simulink model "Hornsea_anant_with_STATCOM (1)"  (R2023b)
settings: Solver=ode1  StartTime=0.0  StopTime=sim_config.Tsim  RelTol=1e-3
undefined symbols (not defined in the file): sim_config
libraries: myLibrary x43, spsThreePhaseVIMeasurementLib x22, spsPower3phInstantaneousLib x11, spspowerguiLib x1
settings Model: Creator=Josep  LastModifiedBy=Josep

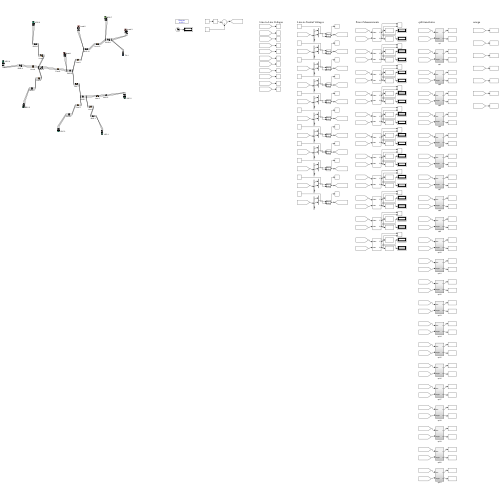
[thumbnail: Simulink's stored preview of the top-level diagram]
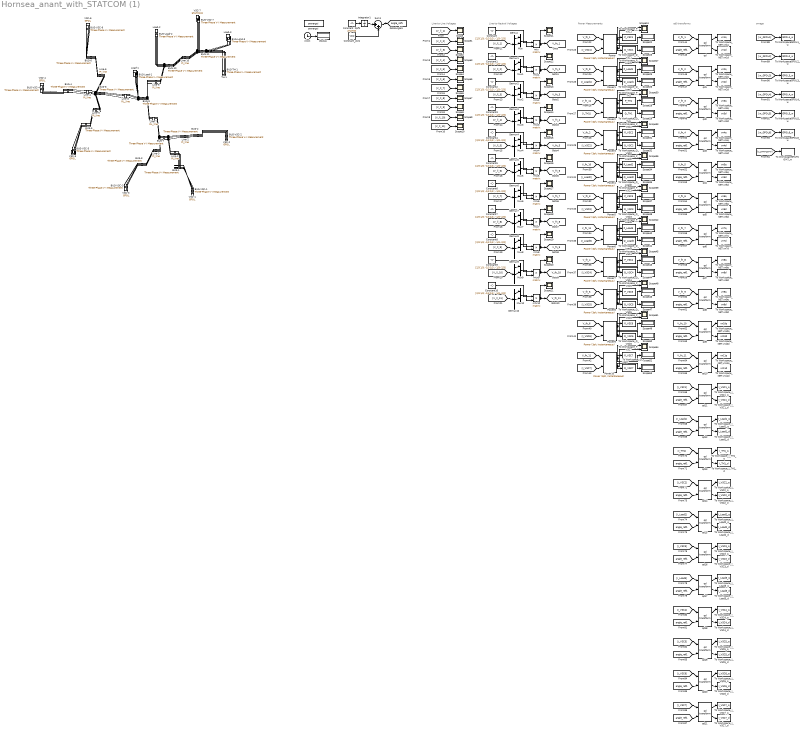
== system Hornsea_anant_with_STATCOM (1) ==
  note: Line-to-Line Voltages
  note: Line-to-Neutral Voltages
  note: Power Measurements
  note: qd0 transforms
  note: omega
  BUS-1 : spsThreePhaseVIMeasurementLib/Three-Phase V-I Measurement  VoltageMeasurement=phase-to-phase  SetLabelV=on  LabelV=V_ll_1  Vpu=off  VpuLL=off  CurrentMeasurement=yes  SetLabelI=on  LabelI=I_1  Ipu=off  Pbase=100e6  Vbase=500e3  OutputType=Complex  PhasorSimulation=off  PSBequivalent=0
  BUS-10 : spsThreePhaseVIMeasurementLib/Three-Phase V-I Measurement  VoltageMeasurement=phase-to-phase  SetLabelV=on  LabelV=V_ll_10  Vpu=off  VpuLL=off  CurrentMeasurement=yes  SetLabelI=on  LabelI=I_10  Ipu=off  Pbase=100e6  Vbase=500e3  OutputType=Complex  PhasorSimulation=off  PSBequivalent=0
  BUS-11 : spsThreePhaseVIMeasurementLib/Three-Phase V-I Measurement  VoltageMeasurement=phase-to-phase  SetLabelV=on  LabelV=V_ll_11  Vpu=off  VpuLL=off  CurrentMeasurement=yes  SetLabelI=on  LabelI=I_11  Ipu=off  Pbase=100e6  Vbase=500e3  OutputType=Complex  PhasorSimulation=off  PSBequivalent=0
  BUS-2 : spsThreePhaseVIMeasurementLib/Three-Phase V-I Measurement  VoltageMeasurement=phase-to-phase  SetLabelV=on  LabelV=V_ll_2  Vpu=off  VpuLL=off  CurrentMeasurement=yes  SetLabelI=on  LabelI=I_2  Ipu=off  Pbase=100e6  Vbase=500e3  OutputType=Complex  PhasorSimulation=off  PSBequivalent=0
  BUS-3 : spsThreePhaseVIMeasurementLib/Three-Phase V-I Measurement  VoltageMeasurement=phase-to-phase  SetLabelV=on  LabelV=V_ll_3  Vpu=off  VpuLL=off  CurrentMeasurement=yes  SetLabelI=on  LabelI=I_3  Ipu=off  Pbase=100e6  Vbase=500e3  OutputType=Complex  PhasorSimulation=off  PSBequivalent=0
  BUS-4 : spsThreePhaseVIMeasurementLib/Three-Phase V-I Measurement  VoltageMeasurement=phase-to-phase  SetLabelV=on  LabelV=V_ll_4  Vpu=off  VpuLL=off  CurrentMeasurement=yes  SetLabelI=on  LabelI=I_4  Ipu=off  Pbase=100e6  Vbase=500e3  OutputType=Complex  PhasorSimulation=off  PSBequivalent=0
  BUS-5 : spsThreePhaseVIMeasurementLib/Three-Phase V-I Measurement  VoltageMeasurement=phase-to-phase  SetLabelV=on  LabelV=V_ll_5  Vpu=off  VpuLL=off  CurrentMeasurement=yes  SetLabelI=on  LabelI=I_5  Ipu=off  Pbase=100e6  Vbase=500e3  OutputType=Complex  PhasorSimulation=off  PSBequivalent=0
  BUS-6 : spsThreePhaseVIMeasurementLib/Three-Phase V-I Measurement  VoltageMeasurement=phase-to-phase  SetLabelV=on  LabelV=V_ll_6  Vpu=off  VpuLL=off  CurrentMeasurement=yes  SetLabelI=on  LabelI=I_6  Ipu=off  Pbase=100e6  Vbase=500e3  OutputType=Complex  PhasorSimulation=off  PSBequivalent=0
  BUS-7 : spsThreePhaseVIMeasurementLib/Three-Phase V-I Measurement  VoltageMeasurement=phase-to-phase  SetLabelV=on  LabelV=V_ll_7  Vpu=off  VpuLL=off  CurrentMeasurement=yes  SetLabelI=on  LabelI=I_7  Ipu=off  Pbase=100e6  Vbase=500e3  OutputType=Complex  PhasorSimulation=off  PSBequivalent=0
  BUS-8 : spsThreePhaseVIMeasurementLib/Three-Phase V-I Measurement  VoltageMeasurement=phase-to-phase  SetLabelV=on  LabelV=V_ll_8  Vpu=off  VpuLL=off  CurrentMeasurement=yes  SetLabelI=on  LabelI=I_8  Ipu=off  Pbase=100e6  Vbase=500e3  OutputType=Complex  PhasorSimulation=off  PSBequivalent=0
  BUS-9 : spsThreePhaseVIMeasurementLib/Three-Phase V-I Measurement  VoltageMeasurement=phase-to-phase  SetLabelV=on  LabelV=V_ll_9  Vpu=off  VpuLL=off  CurrentMeasurement=yes  SetLabelI=on  LabelI=I_9  Ipu=off  Pbase=100e6  Vbase=500e3  OutputType=Complex  PhasorSimulation=off  PSBequivalent=0
  BUS-Load-1 : spsThreePhaseVIMeasurementLib/Three-Phase V-I Measurement  VoltageMeasurement=phase-to-phase  SetLabelV=on  LabelV=V_Load_1  Vpu=off  VpuLL=off  CurrentMeasurement=yes  SetLabelI=on  LabelI=I_Load1  Ipu=off  Pbase=100e6  Vbase=500e3  OutputType=Complex  PhasorSimulation=off  PSBequivalent=0
  BUS-Load-2 : spsThreePhaseVIMeasurementLib/Three-Phase V-I Measurement  VoltageMeasurement=phase-to-phase  SetLabelV=on  LabelV=V_Load_2  Vpu=off  VpuLL=off  CurrentMeasurement=yes  SetLabelI=on  LabelI=I_Load2  Ipu=off  Pbase=100e6  Vbase=500e3  OutputType=Complex  PhasorSimulation=off  PSBequivalent=0
  BUS-Load-3 : spsThreePhaseVIMeasurementLib/Three-Phase V-I Measurement  VoltageMeasurement=phase-to-phase  SetLabelV=on  LabelV=V_Load_3  Vpu=off  VpuLL=off  CurrentMeasurement=yes  SetLabelI=on  LabelI=I_Load3  Ipu=off  Pbase=100e6  Vbase=500e3  OutputType=Complex  PhasorSimulation=off  PSBequivalent=0
  BUS-TH-1 : spsThreePhaseVIMeasurementLib/Three-Phase V-I Measurement  VoltageMeasurement=phase-to-phase  SetLabelV=on  LabelV=V_TH_1  Vpu=off  VpuLL=off  CurrentMeasurement=yes  SetLabelI=on  LabelI=I_TH1  Ipu=off  Pbase=100e6  Vbase=500e3  OutputType=Complex  PhasorSimulation=off  PSBequivalent=0
  BUS-VSC-1 : spsThreePhaseVIMeasurementLib/Three-Phase V-I Measurement  VoltageMeasurement=phase-to-phase  SetLabelV=on  LabelV=V_VSC_1  Vpu=off  VpuLL=off  CurrentMeasurement=yes  SetLabelI=on  LabelI=I_VSC1  Ipu=off  Pbase=100e6  Vbase=500e3  OutputType=Complex  PhasorSimulation=off  PSBequivalent=0
  BUS-VSC-2 : spsThreePhaseVIMeasurementLib/Three-Phase V-I Measurement  VoltageMeasurement=phase-to-phase  SetLabelV=on  LabelV=V_VSC_2  Vpu=off  VpuLL=off  CurrentMeasurement=yes  SetLabelI=on  LabelI=I_VSC2  Ipu=off  Pbase=100e6  Vbase=500e3  OutputType=Complex  PhasorSimulation=off  PSBequivalent=0
  BUS-VSC-3 : spsThreePhaseVIMeasurementLib/Three-Phase V-I Measurement  VoltageMeasurement=phase-to-phase  SetLabelV=on  LabelV=V_VSC_3  Vpu=off  VpuLL=off  CurrentMeasurement=yes  SetLabelI=on  LabelI=I_VSC3  Ipu=off  Pbase=100e6  Vbase=500e3  OutputType=Complex  PhasorSimulation=off  PSBequivalent=0
  BUS-VSC-4 : spsThreePhaseVIMeasurementLib/Three-Phase V-I Measurement  VoltageMeasurement=phase-to-phase  SetLabelV=on  LabelV=V_VSC_4  Vpu=off  VpuLL=off  CurrentMeasurement=yes  SetLabelI=on  LabelI=I_VSC4  Ipu=off  Pbase=100e6  Vbase=500e3  OutputType=Complex  PhasorSimulation=off  PSBequivalent=0
  BUS-VSC-5 : spsThreePhaseVIMeasurementLib/Three-Phase V-I Measurement  VoltageMeasurement=phase-to-phase  SetLabelV=on  LabelV=V_VSC_5  Vpu=off  VpuLL=off  CurrentMeasurement=yes  SetLabelI=on  LabelI=I_VSC5  Ipu=off  Pbase=100e6  Vbase=500e3  OutputType=Complex  PhasorSimulation=off  PSBequivalent=0
  BUS-VSC-6 : spsThreePhaseVIMeasurementLib/Three-Phase V-I Measurement  VoltageMeasurement=phase-to-phase  SetLabelV=on  LabelV=V_VSC_6  Vpu=off  VpuLL=off  CurrentMeasurement=yes  SetLabelI=on  LabelI=I_VSC6  Ipu=off  Pbase=100e6  Vbase=500e3  OutputType=Complex  PhasorSimulation=off  PSBequivalent=0
  BUS-VSC-7 : spsThreePhaseVIMeasurementLib/Three-Phase V-I Measurement  VoltageMeasurement=phase-to-phase  SetLabelV=on  LabelV=V_VSC_7  Vpu=off  VpuLL=off  CurrentMeasurement=yes  SetLabelI=on  LabelI=I_VSC7  Ipu=off  Pbase=100e6  Vbase=500e3  OutputType=Complex  PhasorSimulation=off  PSBequivalent=0
  Constant{,1..10} (11 alike) : Constant  Value=[2/3 1/3; -1/3 1/3 ; -1/3 -2/3]
  Constant_2pif1 : Constant  Value=2*pi*50
  Constant_pi21 : Constant  Value=-pi/2
  Demux{,1..10} (11 alike) : Demux  Outputs=3
  Integrator1 : Integrator
  Line-1 : myLibrary/PI_line  T_line_global=T_NET  initLine_global=init_line  num=1  set_C0=ones(1,6)  set_iL0=0
  Line-10 : myLibrary/PI_line  T_line_global=T_NET  initLine_global=init_line  num=10  set_C0=ones(1,6)  set_iL0=0
  Line-2 : myLibrary/PI_line  T_line_global=T_NET  initLine_global=init_line  num=2  set_C0=ones(1,6)  set_iL0=0
  Line-3 : myLibrary/PI_line  T_line_global=T_NET  initLine_global=init_line  num=3  set_C0=ones(1,6)  set_iL0=0
  Line-4 : myLibrary/PI_line  T_line_global=T_NET  initLine_global=init_line  num=4  set_C0=ones(1,6)  set_iL0=0
  Line-5 : myLibrary/PI_line  T_line_global=T_NET  initLine_global=init_line  num=5  set_C0=ones(1,6)  set_iL0=0
  Line-6 : myLibrary/PI_line  T_line_global=T_NET  initLine_global=init_line  num=6  set_C0=ones(1,6)  set_iL0=0
  Line-7 : myLibrary/RL_line  T_line_global=T_NET  initLine_global=init_line  num=7
  Line-8 : myLibrary/RL_line  T_line_global=T_NET  initLine_global=init_line  num=8
  Line-9 : myLibrary/PI_line  T_line_global=T_NET  initLine_global=init_line  num=9  set_C0=ones(1,6)  set_iL0=0
  Load-1 : myLibrary/Load  T_load_global=T_load  initLoad_global=init_load  num=1
  Load-2 : myLibrary/Load  T_load_global=T_load  initLoad_global=init_load  num=2
  Load-3 : myLibrary/Load  T_load_global=T_load  initLoad_global=init_load  num=3
  Mux{,1..10} (11 alike) : Mux  Inputs=2
  Power{,1..10} (11 alike) : spsPower3phInstantaneousLib/Power (3ph, Instantaneous)
  Scope{,1..21} (22 alike) : Scope
  Scope{22..23,25..26,28..29,31..32,34..35,37..38,40..41,43..44,46..47,49..50,52..53} (22 alike) : Display
  Scope{24,27,30,33,36,39,42,45,48,51,54} (11 alike) : Scope  NumInputPorts=2
  Sum1 : Sum  Inputs=|++
  TH-1 : myLibrary/TH  T_TH_global=T_TH  initTH_global=init_TH  num=1
  To WorkspaceGFOL1_w : ToWorkspace  VariableName=GFOL1_w  SampleTime=sim_config.Tsample
  To WorkspaceGFOL2_w : ToWorkspace  VariableName=GFOL2_w  SampleTime=sim_config.Tsample
  To WorkspaceGFOL3_w : ToWorkspace  VariableName=GFOL3_w  SampleTime=sim_config.Tsample
  To WorkspaceGFOL4_w : ToWorkspace  VariableName=GFOL4_w  SampleTime=sim_config.Tsample
  To WorkspaceGFOL5_w : ToWorkspace  VariableName=GFOL5_w  SampleTime=sim_config.Tsample
  To WorkspaceGFOL6_w : ToWorkspace  VariableName=GFOL6_w  SampleTime=sim_config.Tsample
  To WorkspaceSTATCOM7_w : ToWorkspace  VariableName=STATCOM7_w  SampleTime=sim_config.Tsample
  To Workspace_I_Load1_d : ToWorkspace  VariableName=I_Load1_d  SampleTime=sim_config.Tsample
  To Workspace_I_Load1_q : ToWorkspace  VariableName=I_Load1_q  SampleTime=sim_config.Tsample
  To Workspace_I_Load2_d : ToWorkspace  VariableName=I_Load2_d  SampleTime=sim_config.Tsample
  To Workspace_I_Load2_q : ToWorkspace  VariableName=I_Load2_q  SampleTime=sim_config.Tsample
  To Workspace_I_Load3_d : ToWorkspace  VariableName=I_Load3_d  SampleTime=sim_config.Tsample
  To Workspace_I_Load3_q : ToWorkspace  VariableName=I_Load3_q  SampleTime=sim_config.Tsample
  To Workspace_I_TH1_d : ToWorkspace  VariableName=I_TH1_d  SampleTime=sim_config.Tsample
  To Workspace_I_TH1_q : ToWorkspace  VariableName=I_TH1_q  SampleTime=sim_config.Tsample
  To Workspace_I_VSC1_d : ToWorkspace  VariableName=I_VSC1_d  SampleTime=sim_config.Tsample
  To Workspace_I_VSC1_q : ToWorkspace  VariableName=I_VSC1_q  SampleTime=sim_config.Tsample
  To Workspace_I_VSC2_d : ToWorkspace  VariableName=I_VSC2_d  SampleTime=sim_config.Tsample
  To Workspace_I_VSC2_q : ToWorkspace  VariableName=I_VSC2_q  SampleTime=sim_config.Tsample
  To Workspace_I_VSC3_d : ToWorkspace  VariableName=I_VSC3_d  SampleTime=sim_config.Tsample
  To Workspace_I_VSC3_q : ToWorkspace  VariableName=I_VSC3_q  SampleTime=sim_config.Tsample
  To Workspace_I_VSC4_d : ToWorkspace  VariableName=I_VSC4_d  SampleTime=sim_config.Tsample
  To Workspace_I_VSC4_q : ToWorkspace  VariableName=I_VSC4_q  SampleTime=sim_config.Tsample
  To Workspace_I_VSC5_d : ToWorkspace  VariableName=I_VSC5_d  SampleTime=sim_config.Tsample
  To Workspace_I_VSC5_q : ToWorkspace  VariableName=I_VSC5_q  SampleTime=sim_config.Tsample
  To Workspace_I_VSC6_d : ToWorkspace  VariableName=I_VSC6_d  SampleTime=sim_config.Tsample
  To Workspace_I_VSC6_q : ToWorkspace  VariableName=I_VSC6_q  SampleTime=sim_config.Tsample
  To Workspace_I_VSC7_d : ToWorkspace  VariableName=I_VSC7_d  SampleTime=sim_config.Tsample
  To Workspace_I_VSC7_q : ToWorkspace  VariableName=I_VSC7_q  SampleTime=sim_config.Tsample
  To Workspace_NET.vn10d : ToWorkspace  VariableName=vn10d  SampleTime=sim_config.Tsample
  To Workspace_NET.vn10q : ToWorkspace  VariableName=vn10q  SampleTime=sim_config.Tsample
  To Workspace_NET.vn11d : ToWorkspace  VariableName=vn11d  SampleTime=sim_config.Tsample
  To Workspace_NET.vn11q : ToWorkspace  VariableName=vn11q  SampleTime=sim_config.Tsample
  To Workspace_NET.vn1d : ToWorkspace  VariableName=vn1d  SampleTime=sim_config.Tsample
  To Workspace_NET.vn1q : ToWorkspace  VariableName=vn1q  SampleTime=sim_config.Tsample
  To Workspace_NET.vn2d : ToWorkspace  VariableName=vn2d  SampleTime=sim_config.Tsample
  To Workspace_NET.vn2q : ToWorkspace  VariableName=vn2q  SampleTime=sim_config.Tsample
  To Workspace_NET.vn3d : ToWorkspace  VariableName=vn3d  SampleTime=sim_config.Tsample
  To Workspace_NET.vn3q : ToWorkspace  VariableName=vn3q  SampleTime=sim_config.Tsample
  To Workspace_NET.vn4d : ToWorkspace  VariableName=vn4d  SampleTime=sim_config.Tsample
  To Workspace_NET.vn4q : ToWorkspace  VariableName=vn4q  SampleTime=sim_config.Tsample
  To Workspace_NET.vn5d : ToWorkspace  VariableName=vn5d  SampleTime=sim_config.Tsample
  To Workspace_NET.vn5q : ToWorkspace  VariableName=vn5q  SampleTime=sim_config.Tsample
  To Workspace_NET.vn6d : ToWorkspace  VariableName=vn6d  SampleTime=sim_config.Tsample
  To Workspace_NET.vn6q : ToWorkspace  VariableName=vn6q  SampleTime=sim_config.Tsample
  To Workspace_NET.vn7d : ToWorkspace  VariableName=vn7d  SampleTime=sim_config.Tsample
  To Workspace_NET.vn7q : ToWorkspace  VariableName=vn7q  SampleTime=sim_config.Tsample
  To Workspace_NET.vn8d : ToWorkspace  VariableName=vn8d  SampleTime=sim_config.Tsample
  To Workspace_NET.vn8q : ToWorkspace  VariableName=vn8q  SampleTime=sim_config.Tsample
  To Workspace_NET.vn9d : ToWorkspace  VariableName=vn9d  SampleTime=sim_config.Tsample
  To Workspace_NET.vn9q : ToWorkspace  VariableName=vn9q  SampleTime=sim_config.Tsample
  To Workspace_P_Load1 : ToWorkspace  VariableName=P_Load1  SampleTime=sim_config.Tsample
  To Workspace_P_Load2 : ToWorkspace  VariableName=P_Load2  SampleTime=sim_config.Tsample
  To Workspace_P_Load3 : ToWorkspace  VariableName=P_Load3  SampleTime=sim_config.Tsample
  To Workspace_P_TH1 : ToWorkspace  VariableName=P_TH1  SampleTime=sim_config.Tsample
  To Workspace_P_VSC1 : ToWorkspace  VariableName=P_VSC1  SampleTime=sim_config.Tsample
  To Workspace_P_VSC2 : ToWorkspace  VariableName=P_VSC2  SampleTime=sim_config.Tsample
  To Workspace_P_VSC3 : ToWorkspace  VariableName=P_VSC3  SampleTime=sim_config.Tsample
  To Workspace_P_VSC4 : ToWorkspace  VariableName=P_VSC4  SampleTime=sim_config.Tsample
  To Workspace_P_VSC5 : ToWorkspace  VariableName=P_VSC5  SampleTime=sim_config.Tsample
  To Workspace_P_VSC6 : ToWorkspace  VariableName=P_VSC6  SampleTime=sim_config.Tsample
  To Workspace_P_VSC7 : ToWorkspace  VariableName=P_VSC7  SampleTime=sim_config.Tsample
  To Workspace_Q_Load1 : ToWorkspace  VariableName=Q_Load1  SampleTime=sim_config.Tsample
  To Workspace_Q_Load2 : ToWorkspace  VariableName=Q_Load2  SampleTime=sim_config.Tsample
  To Workspace_Q_Load3 : ToWorkspace  VariableName=Q_Load3  SampleTime=sim_config.Tsample
  To Workspace_Q_TH1 : ToWorkspace  VariableName=Q_TH1  SampleTime=sim_config.Tsample
  To Workspace_Q_VSC1 : ToWorkspace  VariableName=Q_VSC1  SampleTime=sim_config.Tsample
  To Workspace_Q_VSC2 : ToWorkspace  VariableName=Q_VSC2  SampleTime=sim_config.Tsample
  To Workspace_Q_VSC3 : ToWorkspace  VariableName=Q_VSC3  SampleTime=sim_config.Tsample
  To Workspace_Q_VSC4 : ToWorkspace  VariableName=Q_VSC4  SampleTime=sim_config.Tsample
  To Workspace_Q_VSC5 : ToWorkspace  VariableName=Q_VSC5  SampleTime=sim_config.Tsample
  To Workspace_Q_VSC6 : ToWorkspace  VariableName=Q_VSC6  SampleTime=sim_config.Tsample
  To Workspace_Q_VSC7 : ToWorkspace  VariableName=Q_VSC7  SampleTime=sim_config.Tsample
  VSC-1 : myLibrary/GFOL  T_VSC_global=T_VSC  initVSC_global=init_VSC  num=1
  VSC-2 : myLibrary/GFOL  T_VSC_global=T_VSC  initVSC_global=init_VSC  num=2
  VSC-3 : myLibrary/GFOL  T_VSC_global=T_VSC  initVSC_global=init_VSC  num=3
  VSC-4 : myLibrary/GFOL  T_VSC_global=T_VSC  initVSC_global=init_VSC  num=4
  VSC-5 : myLibrary/GFOL  T_VSC_global=T_VSC  initVSC_global=init_VSC  num=5
  VSC-6 : myLibrary/GFOL  T_VSC_global=T_VSC  initVSC_global=init_VSC  num=6
  VSC-7 : myLibrary/STATCOM  T_VSC_global=T_VSC  initVSC_global=init_VSC  num=7
  clock : Clock
  display : Display
  mtx{,1..10} (11 alike) : Product  Multiplication=Matrix(*)
  powergui : spspowerguiLib/powergui  Priority=1  SimulationMode=Discrete  SampleTime=sim_config.Ts  frequency=60  Iterations=50  frequencyindice=60  Pbase=100e6  ErrMax=1e-4  UnitsV=kV  UnitsW=MW  buscounter=0  FunctionMessages=off  echomessages=off  EnableUseOfTLC=off  CurrentSourceSwitches=off  DisableSnubberDevices=off  DisableRonSwitches=off  DisableVfSwitches=off  DisplayEquations=off  AutomaticDiscreteSolvers=off  SolverType=Tustin/Backward Euler (TBE)  Interpol=off  ExternalGateDelay=off  methode=off  Ts=100  x0status=blocks  SPID=on  SwTol=0  HookPort=off  NonlinearTolerance=1e-4  nMaxIteration=100  ContinueOnMaxIteration=off  RestoreLinks=warning  ResistiveCurrentMeasurement=off  Frange=[0:2:500]  Ylog=off  Xlog=on  ShowGrid=off  save=off  variable=ZData  structure=0  ZoomFFT=off  StartTime=0.0  cycles=1  DisplayStyle=1  fundamental=60  FreqAxis=off  MaxFrequency=1000  frequencyindicesteady=1  RmsSteady=1  display=off
  qd{,1..21} (22 alike) : myLibrary/qd transform  SystemSampleTime=-1  VariantActivationTime=update diagram  AllowFlexibleInterface=on  Latency=0  AutoFrameSizeCalculation=off
  tag scope: V_fn_10=global, V_fn_11=global, V_fn_1=global, V_fn_2=global, V_fn_3=global, V_fn_4=global, V_fn_5=global, V_fn_6=global, V_fn_7=global, V_fn_8=global, V_fn_9=global, angle_ref1=global
  wires:
  clock/1 -> display/1
  Constant_2pif1/1 -> Integrator1/1
  Integrator1/1 -> Sum1/1
  Constant_pi21/1 -> Sum1/2
  Sum1/1 -> [angle_ref1]
  [V_ll_1] -> Scope/1
  [V_ll_2] -> Scope1/1
  [V_ll_3] -> Scope2/1
  [V_ll_4] -> Scope3/1
  [V_ll_5] -> Scope4/1
  [V_ll_6] -> Scope5/1
  [V_ll_7] -> Scope6/1
  [V_ll_8] -> Scope7/1
  [V_ll_9] -> Scope8/1
  [V_ll_10] -> Scope9/1
  [V_ll_11] -> Scope10/1
  [V_ll_1] -> Demux/1
  Demux/1 -> Mux/1
  Demux/2 -> Mux/2
  Mux/1 -> mtx/2
  Constant/1 -> mtx/1
  mtx/1 -> [V_fn_1], Scope11/1
  [V_ll_2] -> Demux1/1
  Demux1/1 -> Mux1/1
  Demux1/2 -> Mux1/2
  Mux1/1 -> mtx1/2
  Constant1/1 -> mtx1/1
  mtx1/1 -> [V_fn_2], Scope12/1
  [V_ll_3] -> Demux2/1
  Demux2/1 -> Mux2/1
  Demux2/2 -> Mux2/2
  Mux2/1 -> mtx2/2
  Constant2/1 -> mtx2/1
  mtx2/1 -> [V_fn_3], Scope13/1
  [V_ll_4] -> Demux3/1
  Demux3/1 -> Mux3/1
  Demux3/2 -> Mux3/2
  Mux3/1 -> mtx3/2
  Constant3/1 -> mtx3/1
  mtx3/1 -> [V_fn_4], Scope14/1
  [V_ll_5] -> Demux4/1
  Demux4/1 -> Mux4/1
  Demux4/2 -> Mux4/2
  Mux4/1 -> mtx4/2
  Constant4/1 -> mtx4/1
  mtx4/1 -> [V_fn_5], Scope15/1
  [V_ll_6] -> Demux5/1
  Demux5/1 -> Mux5/1
  Demux5/2 -> Mux5/2
  Mux5/1 -> mtx5/2
  Constant5/1 -> mtx5/1
  mtx5/1 -> [V_fn_6], Scope16/1
  [V_ll_7] -> Demux6/1
  Demux6/1 -> Mux6/1
  Demux6/2 -> Mux6/2
  Mux6/1 -> mtx6/2
  Constant6/1 -> mtx6/1
  mtx6/1 -> [V_fn_7], Scope17/1
  [V_ll_8] -> Demux7/1
  Demux7/1 -> Mux7/1
  Demux7/2 -> Mux7/2
  Mux7/1 -> mtx7/2
  Constant7/1 -> mtx7/1
  mtx7/1 -> [V_fn_8], Scope18/1
  [V_ll_9] -> Demux8/1
  Demux8/1 -> Mux8/1
  Demux8/2 -> Mux8/2
  Mux8/1 -> mtx8/2
  Constant8/1 -> mtx8/1
  mtx8/1 -> [V_fn_9], Scope19/1
  [V_ll_10] -> Demux9/1
  Demux9/1 -> Mux9/1
  Demux9/2 -> Mux9/2
  Mux9/1 -> mtx9/2
  Constant9/1 -> mtx9/1
  mtx9/1 -> [V_fn_10], Scope20/1
  [V_ll_11] -> Demux10/1
  Demux10/1 -> Mux10/1
  Demux10/2 -> Mux10/2
  Mux10/1 -> mtx10/2
  Constant10/1 -> mtx10/1
  mtx10/1 -> [V_fn_11], Scope21/1
  [V_fn_1] -> Power/1
  [I_VSC1] -> Power/2
  Power/1 -> To Workspace_P_VSC1/1, Scope22/1, Scope24/1
  Power/2 -> To Workspace_Q_VSC1/1, Scope23/1, Scope24/2
  [V_fn_9] -> Power1/1
  [I_Load1] -> Power1/2
  Power1/1 -> To Workspace_P_Load1/1, Scope25/1, Scope27/1
  Power1/2 -> To Workspace_Q_Load1/1, Scope26/1, Scope27/2
  [V_fn_11] -> Power2/1
  [I_TH1] -> Power2/2
  Power2/1 -> To Workspace_P_TH1/1, Scope28/1, Scope30/1
  Power2/2 -> To Workspace_Q_TH1/1, Scope29/1, Scope30/2
  [V_fn_2] -> Power3/1
  [I_VSC2] -> Power3/2
  Power3/1 -> To Workspace_P_VSC2/1, Scope31/1, Scope33/1
  Power3/2 -> To Workspace_Q_VSC2/1, Scope32/1, Scope33/2
  [V_fn_10] -> Power4/1
  [I_Load2] -> Power4/2
  Power4/1 -> To Workspace_P_Load2/1, Scope34/1, Scope36/1
  Power4/2 -> To Workspace_Q_Load2/1, Scope35/1, Scope36/2
  [V_fn_3] -> Power5/1
  [I_VSC3] -> Power5/2
  Power5/1 -> To Workspace_P_VSC3/1, Scope37/1, Scope39/1
  Power5/2 -> To Workspace_Q_VSC3/1, Scope38/1, Scope39/2
  [V_fn_11] -> Power6/1
  [I_Load3] -> Power6/2
  Power6/1 -> To Workspace_P_Load3/1, Scope40/1, Scope42/1
  Power6/2 -> To Workspace_Q_Load3/1, Scope41/1, Scope42/2
  [V_fn_4] -> Power7/1
  [I_VSC4] -> Power7/2
  Power7/1 -> To Workspace_P_VSC4/1, Scope43/1, Scope45/1
  Power7/2 -> To Workspace_Q_VSC4/1, Scope44/1, Scope45/2
  [V_fn_5] -> Power8/1
  [I_VSC5] -> Power8/2
  Power8/1 -> To Workspace_P_VSC5/1, Scope46/1, Scope48/1
  Power8/2 -> To Workspace_Q_VSC5/1, Scope47/1, Scope48/2
  [V_fn_6] -> Power9/1
  [I_VSC6] -> Power9/2
  Power9/1 -> To Workspace_P_VSC6/1, Scope49/1, Scope51/1
  Power9/2 -> To Workspace_Q_VSC6/1, Scope50/1, Scope51/2
  [V_fn_11] -> Power10/1
  [I_VSC7] -> Power10/2
  Power10/1 -> To Workspace_P_VSC7/1, Scope52/1, Scope54/1
  Power10/2 -> To Workspace_Q_VSC7/1, Scope53/1, Scope54/2
  [V_fn_1] -> qd/1
  [angle_ref1] -> qd/2
  qd/1 -> To Workspace_NET.vn1q/1
  qd/2 -> To Workspace_NET.vn1d/1
  [V_fn_2] -> qd1/1
  [angle_ref1] -> qd1/2
  qd1/1 -> To Workspace_NET.vn2q/1
  qd1/2 -> To Workspace_NET.vn2d/1
  [V_fn_3] -> qd2/1
  [angle_ref1] -> qd2/2
  qd2/1 -> To Workspace_NET.vn3q/1
  qd2/2 -> To Workspace_NET.vn3d/1
  [V_fn_4] -> qd3/1
  [angle_ref1] -> qd3/2
  qd3/1 -> To Workspace_NET.vn4q/1
  qd3/2 -> To Workspace_NET.vn4d/1
  [V_fn_5] -> qd4/1
  [angle_ref1] -> qd4/2
  qd4/1 -> To Workspace_NET.vn5q/1
  qd4/2 -> To Workspace_NET.vn5d/1
  [V_fn_6] -> qd5/1
  [angle_ref1] -> qd5/2
  qd5/1 -> To Workspace_NET.vn6q/1
  qd5/2 -> To Workspace_NET.vn6d/1
  [V_fn_7] -> qd6/1
  [angle_ref1] -> qd6/2
  qd6/1 -> To Workspace_NET.vn7q/1
  qd6/2 -> To Workspace_NET.vn7d/1
  [V_fn_8] -> qd7/1
  [angle_ref1] -> qd7/2
  qd7/1 -> To Workspace_NET.vn8q/1
  qd7/2 -> To Workspace_NET.vn8d/1
  [V_fn_9] -> qd8/1
  [angle_ref1] -> qd8/2
  qd8/1 -> To Workspace_NET.vn9q/1
  qd8/2 -> To Workspace_NET.vn9d/1
  [V_fn_10] -> qd9/1
  [angle_ref1] -> qd9/2
  qd9/1 -> To Workspace_NET.vn10q/1
  qd9/2 -> To Workspace_NET.vn10d/1
  [V_fn_11] -> qd10/1
  [angle_ref1] -> qd10/2
  qd10/1 -> To Workspace_NET.vn11q/1
  qd10/2 -> To Workspace_NET.vn11d/1
  [I_VSC1] -> qd11/1
  [angle_ref1] -> qd11/2
  qd11/1 -> To Workspace_I_VSC1_q/1
  qd11/2 -> To Workspace_I_VSC1_d/1
  [I_Load1] -> qd12/1
  [angle_ref1] -> qd12/2
  qd12/1 -> To Workspace_I_Load1_q/1
  qd12/2 -> To Workspace_I_Load1_d/1
  [I_TH1] -> qd13/1
  [angle_ref1] -> qd13/2
  qd13/1 -> To Workspace_I_TH1_q/1
  qd13/2 -> To Workspace_I_TH1_d/1
  [I_VSC2] -> qd14/1
  [angle_ref1] -> qd14/2
  qd14/1 -> To Workspace_I_VSC2_q/1
  qd14/2 -> To Workspace_I_VSC2_d/1
  [I_Load2] -> qd15/1
  [angle_ref1] -> qd15/2
  qd15/1 -> To Workspace_I_Load2_q/1
  qd15/2 -> To Workspace_I_Load2_d/1
  [I_VSC3] -> qd16/1
  [angle_ref1] -> qd16/2
  qd16/1 -> To Workspace_I_VSC3_q/1
  qd16/2 -> To Workspace_I_VSC3_d/1
  [I_Load3] -> qd17/1
  [angle_ref1] -> qd17/2
  qd17/1 -> To Workspace_I_Load3_q/1
  qd17/2 -> To Workspace_I_Load3_d/1
  [I_VSC4] -> qd18/1
  [angle_ref1] -> qd18/2
  qd18/1 -> To Workspace_I_VSC4_q/1
  qd18/2 -> To Workspace_I_VSC4_d/1
  [I_VSC5] -> qd19/1
  [angle_ref1] -> qd19/2
  qd19/1 -> To Workspace_I_VSC5_q/1
  qd19/2 -> To Workspace_I_VSC5_d/1
  [I_VSC6] -> qd20/1
  [angle_ref1] -> qd20/2
  qd20/1 -> To Workspace_I_VSC6_q/1
  qd20/2 -> To Workspace_I_VSC6_d/1
  [I_VSC7] -> qd21/1
  [angle_ref1] -> qd21/2
  qd21/1 -> To Workspace_I_VSC7_q/1
  qd21/2 -> To Workspace_I_VSC7_d/1
  [w_GFOL1] -> To WorkspaceGFOL1_w/1
  [w_GFOL2] -> To WorkspaceGFOL2_w/1
  [w_GFOL3] -> To WorkspaceGFOL3_w/1
  [w_GFOL4] -> To WorkspaceGFOL4_w/1
  [w_GFOL5] -> To WorkspaceGFOL5_w/1
  [w_GFOL6] -> To WorkspaceGFOL6_w/1
  [w_STATCOM7] -> To WorkspaceSTATCOM7_w/1
  connections:
  Line-7/LConn1 -- BUS-7/LConn1 -- Line-3/RConn1
  Line-7/LConn2 -- BUS-7/LConn2 -- Line-3/RConn2
  Line-7/LConn3 -- BUS-7/LConn3 -- Line-3/RConn3
  BUS-9/RConn1 -- Line-7/RConn1 -- Line-9/LConn1
  BUS-9/RConn2 -- Line-7/RConn2 -- Line-9/LConn2
  BUS-9/RConn3 -- Line-7/RConn3 -- Line-9/LConn3
  BUS-Load-1/LConn1 -- BUS-9/LConn1 -- Line-8/RConn1
  BUS-Load-1/LConn2 -- BUS-9/LConn2 -- Line-8/RConn2
  BUS-Load-1/LConn3 -- BUS-9/LConn3 -- Line-8/RConn3
  BUS-Load-1/RConn1 -- Load-1/LConn1
  BUS-Load-1/RConn2 -- Load-1/LConn2
  BUS-Load-1/RConn3 -- Load-1/LConn3
  BUS-10/LConn1 -- Line-9/RConn1 -- BUS-Load-2/LConn1
  BUS-10/LConn2 -- Line-9/RConn2 -- BUS-Load-2/LConn2
  BUS-10/LConn3 -- Line-9/RConn3 -- BUS-Load-2/LConn3
  BUS-Load-2/RConn1 -- Load-2/LConn1
  BUS-Load-2/RConn2 -- Load-2/LConn2
  BUS-Load-2/RConn3 -- Load-2/LConn3
  BUS-10/RConn1 -- Line-10/LConn1
  BUS-10/RConn2 -- Line-10/LConn2
  BUS-10/RConn3 -- Line-10/LConn3
  BUS-11/LConn1 -- Line-10/RConn1 -- BUS-VSC-7/RConn1
  BUS-11/LConn2 -- Line-10/RConn2 -- BUS-VSC-7/RConn2
  BUS-11/LConn3 -- Line-10/RConn3 -- BUS-VSC-7/RConn3
  BUS-Load-3/LConn1 -- BUS-11/RConn1 -- BUS-TH-1/RConn1
  BUS-Load-3/LConn2 -- BUS-11/RConn2 -- BUS-TH-1/RConn2
  BUS-Load-3/LConn3 -- BUS-11/RConn3 -- BUS-TH-1/RConn3
  BUS-Load-3/RConn1 -- Load-3/LConn1
  BUS-Load-3/RConn2 -- Load-3/LConn2
  BUS-Load-3/RConn3 -- Load-3/LConn3
  BUS-TH-1/LConn1 -- TH-1/RConn1
  BUS-TH-1/LConn2 -- TH-1/RConn2
  BUS-TH-1/LConn3 -- TH-1/RConn3
  BUS-VSC-7/LConn1 -- VSC-7/RConn1
  BUS-VSC-7/LConn2 -- VSC-7/RConn2
  BUS-VSC-7/LConn3 -- VSC-7/RConn3
  BUS-8/RConn1 -- Line-8/LConn1
  BUS-8/RConn2 -- Line-8/LConn2
  BUS-8/RConn3 -- Line-8/LConn3
  BUS-4/RConn1 -- Line-4/LConn1
  BUS-4/RConn2 -- Line-4/LConn2
  BUS-4/RConn3 -- Line-4/LConn3
  Line-4/RConn1 -- Line-5/RConn1 -- BUS-8/LConn1 -- Line-6/RConn1
  Line-4/RConn2 -- Line-5/RConn2 -- BUS-8/LConn2 -- Line-6/RConn2
  Line-4/RConn3 -- Line-5/RConn3 -- BUS-8/LConn3 -- Line-6/RConn3
  BUS-4/LConn1 -- BUS-VSC-4/RConn1
  BUS-4/LConn2 -- BUS-VSC-4/RConn2
  BUS-4/LConn3 -- BUS-VSC-4/RConn3
  BUS-VSC-4/LConn1 -- VSC-4/RConn1
  BUS-VSC-4/LConn2 -- VSC-4/RConn2
  BUS-VSC-4/LConn3 -- VSC-4/RConn3
  BUS-5/RConn1 -- Line-5/LConn1
  BUS-5/RConn2 -- Line-5/LConn2
  BUS-5/RConn3 -- Line-5/LConn3
  BUS-5/LConn1 -- BUS-VSC-5/RConn1
  BUS-5/LConn2 -- BUS-VSC-5/RConn2
  BUS-5/LConn3 -- BUS-VSC-5/RConn3
  BUS-VSC-5/LConn1 -- VSC-5/RConn1
  BUS-VSC-5/LConn2 -- VSC-5/RConn2
  BUS-VSC-5/LConn3 -- VSC-5/RConn3
  BUS-6/RConn1 -- Line-6/LConn1
  BUS-6/RConn2 -- Line-6/LConn2
  BUS-6/RConn3 -- Line-6/LConn3
  BUS-6/LConn1 -- BUS-VSC-6/RConn1
  BUS-6/LConn2 -- BUS-VSC-6/RConn2
  BUS-6/LConn3 -- BUS-VSC-6/RConn3
  BUS-VSC-6/LConn1 -- VSC-6/RConn1
  BUS-VSC-6/LConn2 -- VSC-6/RConn2
  BUS-VSC-6/LConn3 -- VSC-6/RConn3
  BUS-1/LConn1 -- Line-1/LConn1
  BUS-1/LConn2 -- Line-1/LConn2
  BUS-1/LConn3 -- Line-1/LConn3
  BUS-7/RConn1 -- Line-1/RConn1 -- Line-2/RConn1
  BUS-7/RConn2 -- Line-1/RConn2 -- Line-2/RConn2
  BUS-7/RConn3 -- Line-1/RConn3 -- Line-2/RConn3
  BUS-1/RConn1 -- BUS-VSC-1/RConn1
  BUS-1/RConn2 -- BUS-VSC-1/RConn2
  BUS-1/RConn3 -- BUS-VSC-1/RConn3
  BUS-VSC-1/LConn1 -- VSC-1/RConn1
  BUS-VSC-1/LConn2 -- VSC-1/RConn2
  BUS-VSC-1/LConn3 -- VSC-1/RConn3
  BUS-2/LConn1 -- Line-2/LConn1
  BUS-2/LConn2 -- Line-2/LConn2
  BUS-2/LConn3 -- Line-2/LConn3
  BUS-2/RConn1 -- BUS-VSC-2/RConn1
  BUS-2/RConn2 -- BUS-VSC-2/RConn2
  BUS-2/RConn3 -- BUS-VSC-2/RConn3
  BUS-VSC-2/LConn1 -- VSC-2/RConn1
  BUS-VSC-2/LConn2 -- VSC-2/RConn2
  BUS-VSC-2/LConn3 -- VSC-2/RConn3
  BUS-3/RConn1 -- Line-3/LConn1
  BUS-3/RConn2 -- Line-3/LConn2
  BUS-3/RConn3 -- Line-3/LConn3
  BUS-3/LConn1 -- BUS-VSC-3/RConn1
  BUS-3/LConn2 -- BUS-VSC-3/RConn2
  BUS-3/LConn3 -- BUS-VSC-3/RConn3
  BUS-VSC-3/LConn1 -- VSC-3/RConn1
  BUS-VSC-3/LConn2 -- VSC-3/RConn2
  BUS-VSC-3/LConn3 -- VSC-3/RConn3
